simulink model "check"  (R2015a)
settings: Solver=ode45  StartTime=0.0  StopTime=10.0  RelTol=1e-3
undefined symbols (not defined in the file or in its folder): gray
libraries: visionsinks x2, visionsources x1, neural x1, visiongeotforms x1
settings Model: Creator=Jithendra HS  LastModifiedBy=Jithendra HS

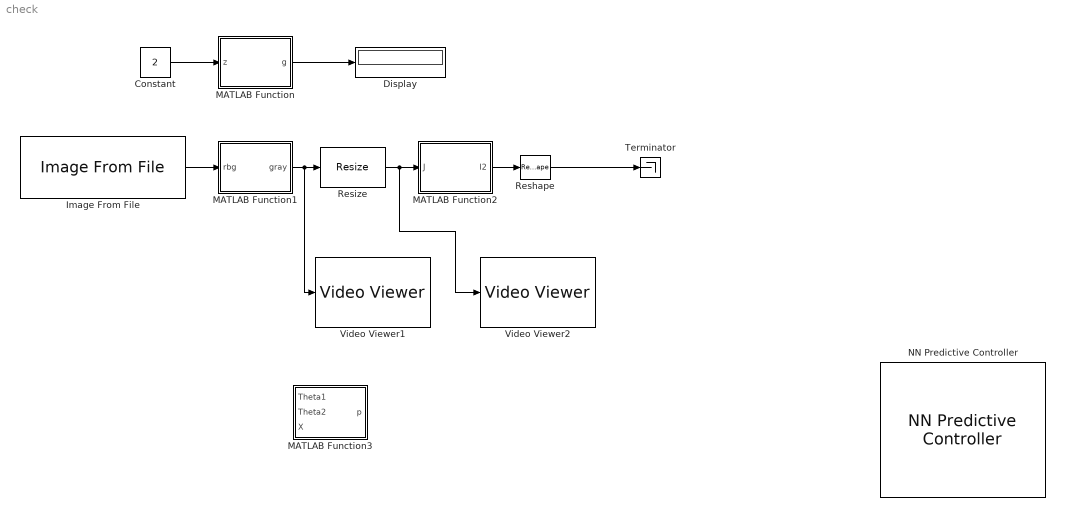
== system check ==
  Constant : Constant  Value=2
  Display : Display
  Image From File : visionsources/Image From File  Tag=vipblks_nd  FileName=C:\Users\Jithendra HS\Documents\project\dsp project\four.JPG  imagePorts=One multidimensional signal  Ts=inf  ImageDataType=Inherit from input image  Signed=on  WordLength=16  sdImageDataType=uint(8)  FractionLengthMode=User-defined  FractionLength=15  OutPortLabels=R|G|B
  MATLAB Function : MATLAB Function  TreatAsAtomicUnit=on
  MATLAB Function1 : MATLAB Function  TreatAsAtomicUnit=on
  MATLAB Function2 : MATLAB Function  TreatAsAtomicUnit=on
  MATLAB Function3 : MATLAB Function  TreatAsAtomicUnit=on
  NN Predictive Controller : neural/Control Systems/NN Predictive Controller  epochs=[]  minp=[]  maxp=[]  mint=[]  maxt=[]  Normalize=[]  IW=[]  LW1_2=[]  LW2_1=[]  B1=[]  B2=[]  max_i_int=[]  min_i_int=[]  limit_output=[]  max_output=[]  min_output=[]  Use_Previous_Weights=[]  N2=[]  Nu=[]  Ts=[]  rho=[]  alpha=[]  csrchfun=csrchbac  maxiter=[]  S1=[]  Ni=[]  Nj=[]  sim_file=0  trainfun=trainlm  Use_validation=[]  Use_Testing=[]  max_i=[]  min_i=[]  sam_training=[]
  Reshape : Reshape  OutputDimensionality=Row vector (2-D)  OutputDimensions=[1,400]
  Resize : visiongeotforms/Resize  specify=Number of output rows and columns  rfactor=[20 20]  outCols=25  outRows=25  outRowsCols=[20 20]  interp_method=Bilinear  antialias=on  useROI=off  roiFlag=off  prodOutputMode=Binary point scaling  prodOutputWordLength=32  prodOutputFracLength=10  roundingMode=Nearest  overflowMode=on
  Terminator : Terminator
  Video Viewer1 : visionsinks/Video Viewer  inputType=Obsolete7b  imagePorts=One multidimensional signal  useColorMap=off  colormapValue=gray(256)  specRange=off  minInputVal=0  maxInputVal=255  FigPos=[1 1028 525 247]  AxisZoom=on  trueSizedOnce=off  OpenAtMdlStart=on  DefaultConfigurationName=vipscopes.VideoViewerScopeCfg
  Video Viewer2 : visionsinks/Video Viewer  inputType=Obsolete7b  imagePorts=One multidimensional signal  useColorMap=off  colormapValue=gray(256)  specRange=off  minInputVal=0  maxInputVal=255  FigPos=[79 802 465 293]  AxisZoom=on  trueSizedOnce=off  OpenAtMdlStart=on  DefaultConfigurationName=vipscopes.VideoViewerScopeCfg
  wires:
  Constant/1 -> MATLAB Function/1(z)
  MATLAB Function/1(g) -> Display/1
  Image From File/1 -> MATLAB Function1/1(rbg)
  MATLAB Function1/1(gray) -> Video Viewer1/1, Resize/1
  Resize/1 -> Video Viewer2/1, MATLAB Function2/1(J)
  MATLAB Function2/1(I2) -> Reshape/1
  Reshape/1 -> Terminator/1

== matlab function check/MATLAB Function1 ==
  data: rbg input; gray output
function gray = fcn(rbg)
%#codegen
gray=rgb2gray(rbg);
end

== matlab function check/MATLAB Function ==
  data: z input; g output
function g = fcn(z)
%#codegen

g = 1.0 ./ (1.0 + exp(-z));
end

== matlab function check/MATLAB Function2 ==
  data: J input; I2 output
function I2 = fcn(J)
%#codegen

I2 = im2double(J);
end

== matlab function check/MATLAB Function3 ==
  data: Theta1 input; p output; Theta2 input; X input
function p = fcn(Theta1,Theta2,X)
%#codegen

m = size(X, 1);
num_labels = size(Theta2, 1);

p = zeros(size(X, 1), 1);


a1 = [ones(m, 1) X];
z2 = a1*Theta1';
a2 = [ones(size(z2, 1), 1) sigmoid(z2)];
z3 = a2*Theta2';
a3 = sigmoid(z3);

[p_max, p] = max(a3, [], 2);

end
